simulink model "ChiefMaster_TTC580"  (R2022b)
settings: Solver=FixedStepAuto  StartTime=0.0  StopTime=10  FixedStep=0.01  RelTol=1e-3
values from neighbouring files (symbols this model uses):
  BattBox1_No = single(1)    [Parameters.m]
  BattBox2_No = single(2)    [Parameters.m]
  BattBox3_No = single(3)    [Parameters.m]
  CurrentLB = single(-3)    [Parameters.m]
  CurrentReductionConstant_Lvl0 = single(0.03)    [Parameters.m]
  CurrentReductionConstant_Lvl1 = single(0.05)    [Parameters.m]
  CurrentReductionConstant_Lvl2 = single(0.07)    [Parameters.m]
  CurrentReductionConstant_Lvl3 = single(0.1)    [Parameters.m]
  CurrentUB = single(3)    [Parameters.m]
  DCHV_Minus_In_Delay_ms = single(500)    [Parameters.m]
  FL_sHVC_CellBalanceVoltage_mV = single(3500)    [Parameters.m]
  FL_sInrushCurrent_dividebyzero = single(0.00001)    [Parameters.m]
  FL_u8HMI_BuzzerTimer = uint8(3)    [Parameters.m]
  IP_boActValue = true    [Parameters.m]
  IP_boDeactValue = false    [Parameters.m]
  IP_boInitValue = false    [Parameters.m]
  IP_s_LB = 18000    [Parameters.m]
  IP_s_UB = 22000    [Parameters.m]
  IP_sBatt1_ChargeCurrentMax_Factor = single(0.1)    [Parameters.m]
  IP_sBatt1_ChargeCurrentMax_LB = single(0)    [Parameters.m]
  IP_sBatt1_ChargeCurrentMax_Offset = single(0)    [Parameters.m]
  IP_sBatt1_ChargeCurrentMax_UB = single(6553.5)    [Parameters.m]
  IP_sBatt1_Current_Factor = single(0.1)    [Parameters.m]
  IP_sBatt1_Current_LB = single(-3276.8)    [Parameters.m]
  IP_sBatt1_Current_Offset = single(0)    [Parameters.m]
  IP_sBatt1_Current_UB = single(3276.8)    [Parameters.m]
  IP_sBatt1_DisChargeCurrentMax_Factor = single(0.1)    [Parameters.m]
  IP_sBatt1_DisChargeCurrentMax_LB = single(0)    [Parameters.m]
  IP_sBatt1_DisChargeCurrentMax_Offset = single(0)    [Parameters.m]
  IP_sBatt1_DisChargeCurrentMax_UB = single(6553.5)    [Parameters.m]
  IP_sBatt1_InsulationResistance_Factor = single(5)    [Parameters.m]
  IP_sBatt1_InsulationResistance_LB = single(0)    [Parameters.m]
  IP_sBatt1_InsulationResistance_Offset = single(0)    [Parameters.m]
  IP_sBatt1_InsulationResistance_UB = single(0)    [Parameters.m]
  IP_sBatt1_LiBa_IntResist_mOhm = single(25)    [Parameters.m]
  IP_sBatt1_SOC_Factor = single(1)    [Parameters.m]
  IP_sBatt1_SOC_LB = single(0)    [Parameters.m]
  IP_sBatt1_SOC_Offset = single(0)    [Parameters.m]
  IP_sBatt1_SOC_UB = single(100)    [Parameters.m]
  IP_sBatt1_SOH_Factor = single(1)    [Parameters.m]
  IP_sBatt1_SOH_LB = single(0)    [Parameters.m]
  IP_sBatt1_SOH_Offset = single(0)    [Parameters.m]
  IP_sBatt1_SOH_UB = single(100)    [Parameters.m]
  IP_sBatt1_Ubatt_Factor = single(0.1)    [Parameters.m]
  IP_sBatt1_Ubatt_LB = single(0)    [Parameters.m]
  IP_sBatt1_Ubatt_Offset = single(0)    [Parameters.m]
  IP_sBatt1_Ubatt_UB = single(6553.5)    [Parameters.m]
  IP_sBatt1_UserRi_Factor = single(1)    [Parameters.m]
  IP_sBatt1_UserRi_LB = single(0)    [Parameters.m]
  IP_sBatt1_UserRi_Offset = single(0)    [Parameters.m]
  IP_sBatt1_UserRi_UB = single(255)    [Parameters.m]
  IP_sBatt1_VoltageAtSensor_Factor = single(0.02)    [Parameters.m]
  IP_sBatt1_VoltageAtSensor_LB = single(0)    [Parameters.m]
  IP_sBatt1_VoltageAtSensor_Offset = single(0)    [Parameters.m]
  IP_sBatt1_VoltageAtSensor_UB = single(1310.7)    [Parameters.m]
  IP_sBatt2_LiBa_IntResist_mOhm = single(25)    [Parameters.m]
  IP_sBatt3_LiBa_IntResist_mOhm = single(25)    [Parameters.m]
  IP_sEM_LB = 2000    [Parameters.m]
  IP_sEM_UB = 8000    [Parameters.m]
  IP_sFB_LB = 5000    [Parameters.m]
  IP_sFB_UB = 10000    [Parameters.m]
  IP_sHVIL_LB = 12000    [Parameters.m]
  IP_sHVIL_UB = 15000    [Parameters.m]
  IP_sLoad_Voltage_Factor = single(1)    [Parameters.m]
  IP_sLoad_Voltage_LB = single(0)    [Parameters.m]
  IP_sLoad_Voltage_Offset = single(0)    [Parameters.m]
  IP_sLoad_Voltage_UB = single(65535)    [Parameters.m]
  IP_u8HVIL_Delay_ms = uint8(100)    [Parameters.m]
  IP_u8HW_IN_delay_ms = uint8(100)    [Parameters.m]
  IT_sInsulationSafeValue_kOhm = single(650)    [Parameters.m]
  IT_u8IMD_DelayTime_s = uint8(20)    [Parameters.m]
  MainHV_Minus_In_Delay = single(5)    [Parameters.m]
  MainHV_StatusDelay = single(5)    [Parameters.m]
  NotAvailable_uint16 = single(65535)    [Parameters.m]
  NotAvailable_uint8 = uint8(255)    [Parameters.m]
  OP_boHVIL_Supply = boolean(1)    [Parameters.m]
  SafeCurrentToCloseHV_A = single(5)    [Parameters.m]
  SafeVoltageToCloseHV_V = single(0.5)    [Parameters.m]
  UnexpectedBattChargingFcn_Available = boolean(1)    [Parameters.m]
  Voltage_NA_UB = uint16(65535)    [Parameters.m]
  VoltageSensorAvailableBB1 = boolean(0)    [Parameters.m]
  VoltageSensorAvailableBB2 = boolean(0)    [Parameters.m]
  VoltageSensorAvailableBB3 = boolean(0)    [Parameters.m]
libraries: simulink x184, Library_DataProcessing_v1_1 x167, Library_DataProcessing_v1 x142, libCM x28
(part 9 of 19)

== system ChiefMaster_TTC580/ChiefMaster/Output Processing/CM_OBD/CM_OP_Msg2 ==
  OT_Databus : Inport
  Bus Selector8 : BusSelector  OutputSignals=OT_KL15_Databus.OT_boKL15_BB1,OT_KL15_Databus.OT_boKL15_BB2,OT_KL15_Databus.OT_boKL15_BB3,OT_BDUControl_Databus.OT_boREQ_MainHV_ON_MINUS,OT_BDUControl_Databus.OT_boREQ_MainHV_ON_PLUS,OT_BDUControl_Databus.OT_boREQ_MainHV_ON_Precharge,OT_IMD_Databus.OT_boREQ_IMD_ON_BB1,OT_IMD_Databus.OT_boREQ_IMD_ON_BB2,OT_IMD_Databus.OT_boREQ_IMD_ON_BB3,OT_BatteryBox_HVControl_Databus.OT_boREQ_HV_ON_BB1,OT_BatteryBox_HVControl_Databus.OT_boREQ_HV_ON_BB2,OT_BatteryBox_HVControl_Databus.OT_boREQ_HV_ON_BB3,OT_BDUControl_Databus.OT_boREQ_DC_ON_MINUS,OT_BDUControl_Databus.OT_boREQ_DC_ON_Plus,OT_SystemStatus_Databus.OT_boSS_CabinAlarm,OT_SystemStatus_Databus.OT_boSS_EMSRET_POWER,OT_SystemStatus_Databus.OT_boSS_Resetbutton_LED
  Constant1 : Constant  Value=0  OutDataTypeStr=uint8
  Constant2 : Constant  Value=0  OutDataTypeStr=uint8
  Constant3 : Constant  Value=0  OutDataTypeStr=uint8
  Lib_MultiBit_Concat1 : Library_DataProcessing_v1/Lib_MultiBit_Concat  SystemSampleTime=-1  VariantActivationTime=update diagram  Latency=0  AutoFrameSizeCalculation=off
  Lib_MultiBit_Concat2 : Library_DataProcessing_v1/Lib_MultiBit_Concat  SystemSampleTime=-1  VariantActivationTime=update diagram  Latency=0  AutoFrameSizeCalculation=off
  Lib_MultiBit_Concat7 : Library_DataProcessing_v1/Lib_MultiBit_Concat  SystemSampleTime=-1  VariantActivationTime=update diagram  Latency=0  AutoFrameSizeCalculation=off
  Mux : Mux  Inputs=8
  OP_ChiefMaster_OP_Msg2 : Outport
  wires:
  OT_Databus/1 -> Bus Selector8/1
  Lib_MultiBit_Concat7/1 -> Mux/1
  Bus Selector8/1 -> Lib_MultiBit_Concat7/1  "<OT_boKL15_BB1>"
  Bus Selector8/2 -> Lib_MultiBit_Concat7/2  "<OT_boKL15_BB2>"
  Bus Selector8/3 -> Lib_MultiBit_Concat7/3  "<OT_boKL15_BB3>"
  Bus Selector8/4 -> Lib_MultiBit_Concat7/4  "<OT_boREQ_MainHV_ON_MINUS>"
  Bus Selector8/5 -> Lib_MultiBit_Concat7/5  "<OT_boREQ_MainHV_ON_PLUS>"
  Bus Selector8/6 -> Lib_MultiBit_Concat7/6  "<OT_boREQ_MainHV_ON_Precharge>"
  Constant2/1 -> Mux/7, Mux/6, Mux/4, Mux/5, Mux/8
  Mux/1 -> OP_ChiefMaster_OP_Msg2/1
  Bus Selector8/7 -> Lib_MultiBit_Concat7/7  "<OT_boREQ_IMD_ON_BB1>"
  Bus Selector8/8 -> Lib_MultiBit_Concat7/8  "<OT_boREQ_IMD_ON_BB2>"
  Bus Selector8/9 -> Lib_MultiBit_Concat1/1  "<OT_boREQ_IMD_ON_BB3>"
  Bus Selector8/10 -> Lib_MultiBit_Concat1/2  "<OT_boREQ_HV_ON_BB1>"
  Bus Selector8/11 -> Lib_MultiBit_Concat1/3  "<OT_boREQ_HV_ON_BB2>"
  Bus Selector8/12 -> Lib_MultiBit_Concat1/4  "<OT_boREQ_HV_ON_BB3>"
  Lib_MultiBit_Concat1/1 -> Mux/2
  Bus Selector8/13 -> Lib_MultiBit_Concat1/5  "<OT_boREQ_DC_ON_MINUS>"
  Bus Selector8/14 -> Lib_MultiBit_Concat1/6  "<OT_boREQ_DC_ON_Plus>"
  Bus Selector8/15 -> Lib_MultiBit_Concat2/1  "<OT_boSS_CabinAlarm>"
  Bus Selector8/16 -> Lib_MultiBit_Concat2/2  "<OT_boSS_EMSRET_POWER>"
  Bus Selector8/17 -> Lib_MultiBit_Concat2/3  "<OT_boSS_Resetbutton_LED>"
  Constant1/1 -> Lib_MultiBit_Concat1/7, Lib_MultiBit_Concat1/8
  Constant3/1 -> Lib_MultiBit_Concat2/8, Lib_MultiBit_Concat2/6, Lib_MultiBit_Concat2/4, Lib_MultiBit_Concat2/5, Lib_MultiBit_Concat2/7
  Lib_MultiBit_Concat2/1 -> Mux/3

== system ChiefMaster_TTC580/ChiefMaster/Output Processing/CM_OBD/CM_SystemStatus1_Msg3 ==
  OT_Databus : Inport
  Bus Selector3 : BusSelector  OutputSignals=OT_boCM_Sleep,OT_SystemStatus_Databus.OT_boSS_HVIL_NOK,OT_SystemStatus_Databus.OT_u8SS_ChiefMaster_State,OT_SystemStatus_Databus.OT_u8SS_System_ErrorCode,OT_SystemStatus_Databus.OT_u8SS_System_SD_ErrorCode,OT_SystemStatus_Databus.OT_u8SS_SystemSOC,OT_IMD_Databus.OT_u8_IMD_State_BB1,OT_IMD_Databus.OT_u8_IMD_State_BB2,OT_IMD_Databus.OT_u8_IMD_State_BB3
  Bus Selector5 : BusSelector  OutputSignals=OT_SystemStatus_Databus.OT_boSS_Batt_Warning,OT_SystemStatus_Databus.OT_boSS_Batt_Error,OT_SystemStatus_Databus.OT_boSS_Batt_SDError,OT_SystemStatus_Databus.OT_boSS_System_Error,OT_SystemStatus_Databus.OT_boSS_System_SD,OT_SystemStatus_Databus.OT_boSS_System_ESD,OT_SystemStatus_Databus.OT_boSS_BDU_Reset,FL_Databus.FL_KL15_Databus.FL_boKL15_Disable,FL_Databus.FL_KL15_Databus.FL_boKL15_Reset,FL_Databus.IT_Databus.IT_BatterySignal_Databus.IT_boBMS_HV_ON_BB,FL_Databus.IT_Databus.IT_BatterySignal_Databus.IT_u8BMS_No_of_Battery_Usable,OT_SystemStatus_Databus.OT_u8SS_NumberOfConnectedBatt,OT_SystemStatus_Databus.OT_u8SS_EmergencyStopState
  Constant1 : Constant  Value=0  OutDataTypeStr=uint8
  Constant4 : Constant  Value=0  OutDataTypeStr=uint8
  Extract Bits1 : simulink/Logic and Bit Operations/Extract Bits  bitsToExtract=Range of bits  numBits=8  bitIdxRange=[0 1]  outScalingMode=Treat bit field as an integer
  Extract Bits2 : simulink/Logic and Bit Operations/Extract Bits  bitsToExtract=Range of bits  numBits=8  bitIdxRange=[0 1]  outScalingMode=Treat bit field as an integer
  Extract Bits3 : simulink/Logic and Bit Operations/Extract Bits  bitsToExtract=Range of bits  numBits=8  bitIdxRange=[0 1]  outScalingMode=Treat bit field as an integer
  Extract Bits4 : simulink/Logic and Bit Operations/Extract Bits  bitsToExtract=Range of bits  numBits=8  bitIdxRange=[0 2]  outScalingMode=Treat bit field as an integer
  Extract Bits5 : simulink/Logic and Bit Operations/Extract Bits  bitsToExtract=Range of bits  numBits=8  bitIdxRange=[0 2]  outScalingMode=Treat bit field as an integer
  Extract Bits6 : simulink/Logic and Bit Operations/Extract Bits  bitsToExtract=Range of bits  numBits=8  bitIdxRange=[0 2]  outScalingMode=Treat bit field as an integer
  Lib_MultiBit_Concat{1..4} (4 alike) : Library_DataProcessing_v1/Lib_MultiBit_Concat  SystemSampleTime=-1  VariantActivationTime=update diagram  Latency=0  AutoFrameSizeCalculation=off
  Mux : Mux  Inputs=8
  Subsystem : Subsystem
  OP_ChiefMaster_SS_Msg3 : Outport
  wires:
  Mux/1 -> OP_ChiefMaster_SS_Msg3/1
  Bus Selector5/1 -> Lib_MultiBit_Concat1/1  "<OT_boSS_Batt_Warning>"
  Bus Selector5/2 -> Lib_MultiBit_Concat1/2  "<OT_boSS_Batt_Error>"
  Bus Selector5/3 -> Lib_MultiBit_Concat1/3  "<OT_boSS_Batt_SDError>"
  Bus Selector5/4 -> Lib_MultiBit_Concat1/4  "<OT_boSS_System_Error>"
  Bus Selector5/5 -> Lib_MultiBit_Concat1/5  "<OT_boSS_System_SD>"
  Bus Selector5/6 -> Lib_MultiBit_Concat1/6  "<OT_boSS_System_ESD>"
  Bus Selector5/7 -> Lib_MultiBit_Concat1/7  "<OT_boSS_BDU_Reset>"
  Bus Selector5/12 -> Extract Bits3/1  "<OT_u8SS_NumberOfConnectedBatt>"
  Bus Selector5/13 -> Extract Bits2/1  "<OT_u8SS_EmergencyStopState>"
  Constant4/1 -> Lib_MultiBit_Concat2/6, Lib_MultiBit_Concat2/4, Lib_MultiBit_Concat2/8, Lib_MultiBit_Concat3/4, Lib_MultiBit_Concat3/5, Lib_MultiBit_Concat3/7, Lib_MultiBit_Concat3/8
  Bus Selector5/8 -> Lib_MultiBit_Concat1/8  "<FL_boKL15_Disable>"
  Bus Selector5/9 -> Lib_MultiBit_Concat2/1  "<FL_boKL15_Reset>"
  Lib_MultiBit_Concat1/1 -> Mux/1
  Lib_MultiBit_Concat2/1 -> Mux/2
  Bus Selector5/10 -> Lib_MultiBit_Concat2/2  "<IT_boBMS_HV_ON_BB>"
  Bus Selector5/11 -> Extract Bits1/1  "<IT_u8BMS_No_of_Battery_Usable>"
  Extract Bits1/1 -> Lib_MultiBit_Concat2/3
  Extract Bits3/1 -> Lib_MultiBit_Concat2/5
  Extract Bits2/1 -> Lib_MultiBit_Concat2/7
  Lib_MultiBit_Concat4/1 -> Mux/8
  Bus Selector3/1 -> Lib_MultiBit_Concat3/1  "<OT_boCM_Sleep>"
  Bus Selector3/3 -> Mux/4  "<OT_u8SS_ChiefMaster_State>"
  Lib_MultiBit_Concat3/1 -> Mux/3
  Bus Selector3/4 -> Mux/5  "<OT_u8SS_System_ErrorCode>"
  Bus Selector3/5 -> Mux/6  "<OT_u8SS_System_SD_ErrorCode>"
  Bus Selector3/6 -> Mux/7  "<OT_u8SS_SystemSOC>"
  Bus Selector3/2 -> Lib_MultiBit_Concat3/2  "<OT_boSS_HVIL_NOK>"
  OT_Databus/1 -> Bus Selector5/1, Subsystem/1(IP_DataBus), Bus Selector3/1
  Subsystem/1(FL_boHVC_AllCellBalanced) -> Lib_MultiBit_Concat3/3
  Bus Selector3/7 -> Extract Bits4/1  "<OT_u8_IMD_State_BB1>"
  Bus Selector3/8 -> Extract Bits5/1  "<OT_u8_IMD_State_BB2>"
  Bus Selector3/9 -> Extract Bits6/1  "<OT_u8_IMD_State_BB3>"
  Extract Bits4/1 -> Lib_MultiBit_Concat3/6
  Extract Bits5/1 -> Lib_MultiBit_Concat4/1
  Extract Bits6/1 -> Lib_MultiBit_Concat4/4
  Constant1/1 -> Lib_MultiBit_Concat4/8, Lib_MultiBit_Concat4/7, Lib_MultiBit_Concat4/2, Lib_MultiBit_Concat4/3, Lib_MultiBit_Concat4/5, Lib_MultiBit_Concat4/6

== system ChiefMaster_TTC580/ChiefMaster/Output Processing/CM_OBD/CM_SystemStatus2_Msg4 ==
  OT_Databus : Inport
  Bus Selector3 : BusSelector  OutputSignals=OT_SystemStatus_Databus.OT_sSS_System_Current,OT_SystemStatus_Databus.OT_sSS_SystemVoltage,OT_SystemStatus_Databus.OT_sSS_MaxChargeCurrent,OT_SystemStatus_Databus.OT_sSS_MaxDisChargeCurrent
  Mux1 : Mux  Inputs=8
  Subsystem : Subsystem
  Subsystem1 : Subsystem
  Subsystem2 : Subsystem
  Subsystem3 : Subsystem
  OP_ChiefMaster_SS2_Msg4 : Outport
  wires:
  Subsystem1/1(u8byte_LSB) -> Mux1/3
  Subsystem2/1(u8byte_LSB) -> Mux1/5
  Bus Selector3/4 -> Subsystem3/1(MaxDisChargeCurrent)  "<OT_sSS_MaxDisChargeCurrent>"
  Bus Selector3/1 -> Subsystem/1(System_Current)  "<OT_sSS_System_Current>"
  Subsystem/2(u8byte_MSB) -> Mux1/2
  Subsystem2/2(u8byte_MSB) -> Mux1/6
  Bus Selector3/2 -> Subsystem1/1(System_Voltage)  "<OT_sSS_SystemVoltage>"
  Mux1/1 -> OP_ChiefMaster_SS2_Msg4/1
  Subsystem1/2(u8byte_MSB) -> Mux1/4
  Subsystem3/1(u8byte_LSB) -> Mux1/7
  Bus Selector3/3 -> Subsystem2/1(MaxChargeCurrent)  "<OT_sSS_MaxChargeCurrent>"
  Subsystem3/2(u8byte_MSB) -> Mux1/8
  Subsystem/1(u8byte_LSB) -> Mux1/1
  OT_Databus/1 -> Bus Selector3/1

== system ChiefMaster_TTC580/ChiefMaster/Output Processing/OP_Actia/Subsystem2 ==
  <FL_boREQ_HV_ON_BB1> : Inport
  <FL_boREQ_IMD_ON_BB1> : Inport  Port=2
  Constant15 : Constant  Priority=2915  Value=0
  Constant3 : Constant  Priority=2915  Value=0  OutDataTypeStr=uint8
  Lib_MultiBit_Concat1 : Library_DataProcessing_v1/Lib_MultiBit_Concat  SystemSampleTime=-1  VariantActivationTime=update diagram  Latency=0  AutoFrameSizeCalculation=off
  Mux : Mux  Inputs=8
  OP_Actia_Control_Batt1 : Outport
  wires:
  Constant3/1 -> Mux/7, Mux/6, Mux/5, Mux/4, Mux/3, Mux/2, Mux/8
  Constant15/1 -> Lib_MultiBit_Concat1/7, Lib_MultiBit_Concat1/5, Lib_MultiBit_Concat1/3, Lib_MultiBit_Concat1/4, Lib_MultiBit_Concat1/6, Lib_MultiBit_Concat1/8
  <FL_boREQ_HV_ON_BB1>/1 -> Lib_MultiBit_Concat1/1
  Lib_MultiBit_Concat1/1 -> Mux/1
  Mux/1 -> OP_Actia_Control_Batt1/1
  <FL_boREQ_IMD_ON_BB1>/1 -> Lib_MultiBit_Concat1/2

== system ChiefMaster_TTC580/ChiefMaster/Output Processing/OP_Actia/Subsystem3 ==
  <FL_boREQ_HV_ON_BB2> : Inport
  <FL_boREQ_IMD_ON_BB2> : Inport  Port=2
  Constant1 : Constant  Priority=2915  Value=0
  Constant4 : Constant  Priority=2915  Value=0  OutDataTypeStr=uint8
  Lib_MultiBit_Concat2 : Library_DataProcessing_v1/Lib_MultiBit_Concat  SystemSampleTime=-1  VariantActivationTime=update diagram  Latency=0  AutoFrameSizeCalculation=off
  Mux1 : Mux  Inputs=8
  OP_Actia_Control_Batt2 : Outport
  wires:
  Constant4/1 -> Mux1/8, Mux1/2, Mux1/3, Mux1/4, Mux1/5, Mux1/6, Mux1/7
  Constant1/1 -> Lib_MultiBit_Concat2/8, Lib_MultiBit_Concat2/6, Lib_MultiBit_Concat2/4, Lib_MultiBit_Concat2/3, Lib_MultiBit_Concat2/5, Lib_MultiBit_Concat2/7
  <FL_boREQ_IMD_ON_BB2>/1 -> Lib_MultiBit_Concat2/2
  Lib_MultiBit_Concat2/1 -> Mux1/1
  Mux1/1 -> OP_Actia_Control_Batt2/1
  <FL_boREQ_HV_ON_BB2>/1 -> Lib_MultiBit_Concat2/1

== system ChiefMaster_TTC580/ChiefMaster/Output Processing/OP_Actia/Subsystem4 ==
  <FL_boREQ_HV_ON_BB3> : Inport
  <FL_boREQ_IMD_ON_BB3> : Inport  Port=2
  Constant2 : Constant  Priority=2915  Value=0
  Constant5 : Constant  Priority=2915  Value=0  OutDataTypeStr=uint8
  Lib_MultiBit_Concat3 : Library_DataProcessing_v1/Lib_MultiBit_Concat  SystemSampleTime=-1  VariantActivationTime=update diagram  Latency=0  AutoFrameSizeCalculation=off
  Mux2 : Mux  Inputs=8
  OP_Actia_Control_Batt3 : Outport
  wires:
  <FL_boREQ_IMD_ON_BB3>/1 -> Lib_MultiBit_Concat3/2
  Constant2/1 -> Lib_MultiBit_Concat3/7, Lib_MultiBit_Concat3/5, Lib_MultiBit_Concat3/3, Lib_MultiBit_Concat3/4, Lib_MultiBit_Concat3/6, Lib_MultiBit_Concat3/8
  Constant5/1 -> Mux2/7, Mux2/6, Mux2/5, Mux2/4, Mux2/3, Mux2/2, Mux2/8
  <FL_boREQ_HV_ON_BB3>/1 -> Lib_MultiBit_Concat3/1
  Mux2/1 -> OP_Actia_Control_Batt3/1
  Lib_MultiBit_Concat3/1 -> Mux2/1

== system ChiefMaster_TTC580/ChiefMaster/Output Processing/OP_LiBa/UDC_BMS_OperationRequest1 ==
  OT_Databus : Inport
  Bus Selector1 : BusSelector  OutputSignals=OT_BatteryBox_HVControl_Databus.OT_boREQ_HV_ON_BB1,OT_IMD_Databus.OT_boREQ_IMD_ON_BB1
  Constant{,1..4} (5 alike) : Constant  Value=0  OutDataTypeStr=uint8
  Constant5 : Constant  OutDataTypeStr=uint8
  Data Type Conversion : DataTypeConversion  OutDataTypeStr=uint8  RndMeth=Nearest  SaturateOnIntegerOverflow=off
  Data Type Conversion1 : DataTypeConversion  OutDataTypeStr=uint8  RndMeth=Nearest  SaturateOnIntegerOverflow=off
  Data Type Conversion2 : DataTypeConversion  OutDataTypeStr=uint16  RndMeth=Nearest  SaturateOnIntegerOverflow=off
  Extract Bits : simulink/Logic and Bit Operations/Extract Bits  bitsToExtract=Range of bits  numBits=8  bitIdxRange=[0 1]  outScalingMode=Preserve fixed-point scaling
  Extract Bits1 : simulink/Logic and Bit Operations/Extract Bits  bitsToExtract=Range of bits  numBits=8  bitIdxRange=[0 1]  outScalingMode=Preserve fixed-point scaling
  Extract Bits2 : simulink/Logic and Bit Operations/Extract Bits  bitsToExtract=Range of bits  numBits=8  bitIdxRange=[0 1]  outScalingMode=Preserve fixed-point scaling
  Extract Bits3 : simulink/Logic and Bit Operations/Extract Bits  bitsToExtract=Range of bits  numBits=8  bitIdxRange=[0 7]  outScalingMode=Treat bit field as an integer
  Extract Bits4 : simulink/Logic and Bit Operations/Extract Bits  bitsToExtract=Range of bits  numBits=8  bitIdxRange=[8 15]  outScalingMode=Treat bit field as an integer
  Lib_MultiBit_Concat : Library_DataProcessing_v1_1/Lib_MultiBit_Concat  SystemSampleTime=-1  VariantActivationTime=update diagram  Latency=0  AutoFrameSizeCalculation=off
  Mux : Mux  Inputs=8
  OP_UDC_BMS_OperationRequest : Outport
  wires:
  Mux/1 -> OP_UDC_BMS_OperationRequest/1
  Lib_MultiBit_Concat/1 -> Mux/1
  Constant/1 -> Mux/8, Mux/7, Mux/6, Mux/5, Mux/4
  OT_Databus/1 -> Bus Selector1/1
  Extract Bits/1 -> Lib_MultiBit_Concat/1
  Extract Bits1/1 -> Lib_MultiBit_Concat/3
  Extract Bits2/1 -> Lib_MultiBit_Concat/7
  Constant1/1 -> Lib_MultiBit_Concat/2
  Constant2/1 -> Lib_MultiBit_Concat/6, Lib_MultiBit_Concat/5, Lib_MultiBit_Concat/4
  Constant3/1 -> Lib_MultiBit_Concat/8
  Constant4/1 -> Extract Bits/1
  Constant5/1 -> Extract Bits2/1
  Data Type Conversion/1 -> Mux/2
  Data Type Conversion1/1 -> Mux/3
  Extract Bits4/1 -> Data Type Conversion1/1
  Extract Bits3/1 -> Data Type Conversion/1
  Data Type Conversion2/1 -> Extract Bits4/1, Extract Bits3/1
  Bus Selector1/1 -> Extract Bits1/1  "<OT_boREQ_HV_ON_BB1>"
  Bus Selector1/2 -> Data Type Conversion2/1  "<OT_boREQ_IMD_ON_BB1>"

== system ChiefMaster_TTC580/ChiefMaster/Output Processing/OP_LiBa/UDC_BMS_OperationRequest2 ==
  OT_Databus : Inport
  Bus Selector1 : BusSelector  OutputSignals=OT_BatteryBox_HVControl_Databus.OT_boREQ_HV_ON_BB2,OT_IMD_Databus.OT_boREQ_IMD_ON_BB2
  Constant{,1..4} (5 alike) : Constant  Value=0  OutDataTypeStr=uint8
  Constant5 : Constant  OutDataTypeStr=uint8
  Data Type Conversion : DataTypeConversion  OutDataTypeStr=uint8  RndMeth=Nearest  SaturateOnIntegerOverflow=off
  Data Type Conversion1 : DataTypeConversion  OutDataTypeStr=uint8  RndMeth=Nearest  SaturateOnIntegerOverflow=off
  Data Type Conversion2 : DataTypeConversion  OutDataTypeStr=uint16  RndMeth=Nearest  SaturateOnIntegerOverflow=off
  Extract Bits : simulink/Logic and Bit Operations/Extract Bits  bitsToExtract=Range of bits  numBits=8  bitIdxRange=[0 1]  outScalingMode=Preserve fixed-point scaling
  Extract Bits1 : simulink/Logic and Bit Operations/Extract Bits  bitsToExtract=Range of bits  numBits=8  bitIdxRange=[0 1]  outScalingMode=Preserve fixed-point scaling
  Extract Bits2 : simulink/Logic and Bit Operations/Extract Bits  bitsToExtract=Range of bits  numBits=8  bitIdxRange=[0 1]  outScalingMode=Preserve fixed-point scaling
  Extract Bits3 : simulink/Logic and Bit Operations/Extract Bits  bitsToExtract=Range of bits  numBits=8  bitIdxRange=[0 7]  outScalingMode=Treat bit field as an integer
  Extract Bits4 : simulink/Logic and Bit Operations/Extract Bits  bitsToExtract=Range of bits  numBits=8  bitIdxRange=[8 15]  outScalingMode=Treat bit field as an integer
  Lib_MultiBit_Concat : Library_DataProcessing_v1_1/Lib_MultiBit_Concat  SystemSampleTime=-1  VariantActivationTime=update diagram  Latency=0  AutoFrameSizeCalculation=off
  Mux : Mux  Inputs=8
  OP_UDC_BMS_OperationRequest : Outport
  wires:
  Bus Selector1/2 -> Data Type Conversion2/1  "<OT_boREQ_IMD_ON_BB2>"
  Bus Selector1/1 -> Extract Bits1/1  "<OT_boREQ_HV_ON_BB2>"
  Data Type Conversion2/1 -> Extract Bits3/1, Extract Bits4/1
  Extract Bits3/1 -> Data Type Conversion/1
  Extract Bits4/1 -> Data Type Conversion1/1
  Data Type Conversion1/1 -> Mux/3
  Data Type Conversion/1 -> Mux/2
  Constant5/1 -> Extract Bits2/1
  Constant4/1 -> Extract Bits/1
  Constant3/1 -> Lib_MultiBit_Concat/8
  Constant2/1 -> Lib_MultiBit_Concat/4, Lib_MultiBit_Concat/5, Lib_MultiBit_Concat/6
  Constant1/1 -> Lib_MultiBit_Concat/2
  Extract Bits2/1 -> Lib_MultiBit_Concat/7
  Extract Bits1/1 -> Lib_MultiBit_Concat/3
  Extract Bits/1 -> Lib_MultiBit_Concat/1
  OT_Databus/1 -> Bus Selector1/1
  Constant/1 -> Mux/4, Mux/5, Mux/6, Mux/7, Mux/8
  Lib_MultiBit_Concat/1 -> Mux/1
  Mux/1 -> OP_UDC_BMS_OperationRequest/1

== system ChiefMaster_TTC580/ChiefMaster/Output Processing/OP_LiBa/UDC_BMS_OperationRequest3 ==
  OT_Databus : Inport
  Bus Selector1 : BusSelector  OutputSignals=OT_BatteryBox_HVControl_Databus.OT_boREQ_HV_ON_BB3,OT_IMD_Databus.OT_boREQ_IMD_ON_BB3
  Constant{,1..4} (5 alike) : Constant  Value=0  OutDataTypeStr=uint8
  Constant5 : Constant  OutDataTypeStr=uint8
  Data Type Conversion : DataTypeConversion  OutDataTypeStr=uint8  RndMeth=Nearest  SaturateOnIntegerOverflow=off
  Data Type Conversion1 : DataTypeConversion  OutDataTypeStr=uint8  RndMeth=Nearest  SaturateOnIntegerOverflow=off
  Data Type Conversion2 : DataTypeConversion  OutDataTypeStr=uint16  RndMeth=Nearest  SaturateOnIntegerOverflow=off
  Extract Bits : simulink/Logic and Bit Operations/Extract Bits  bitsToExtract=Range of bits  numBits=8  bitIdxRange=[0 1]  outScalingMode=Preserve fixed-point scaling
  Extract Bits1 : simulink/Logic and Bit Operations/Extract Bits  bitsToExtract=Range of bits  numBits=8  bitIdxRange=[0 1]  outScalingMode=Preserve fixed-point scaling
  Extract Bits2 : simulink/Logic and Bit Operations/Extract Bits  bitsToExtract=Range of bits  numBits=8  bitIdxRange=[0 1]  outScalingMode=Preserve fixed-point scaling
  Extract Bits3 : simulink/Logic and Bit Operations/Extract Bits  bitsToExtract=Range of bits  numBits=8  bitIdxRange=[0 7]  outScalingMode=Treat bit field as an integer
  Extract Bits4 : simulink/Logic and Bit Operations/Extract Bits  bitsToExtract=Range of bits  numBits=8  bitIdxRange=[8 15]  outScalingMode=Treat bit field as an integer
  Lib_MultiBit_Concat : Library_DataProcessing_v1_1/Lib_MultiBit_Concat  SystemSampleTime=-1  VariantActivationTime=update diagram  Latency=0  AutoFrameSizeCalculation=off
  Mux : Mux  Inputs=8
  OP_UDC_BMS_OperationRequest : Outport
  wires:
  Mux/1 -> OP_UDC_BMS_OperationRequest/1
  Lib_MultiBit_Concat/1 -> Mux/1
  Constant/1 -> Mux/8, Mux/7, Mux/6, Mux/5, Mux/4
  OT_Databus/1 -> Bus Selector1/1
  Extract Bits/1 -> Lib_MultiBit_Concat/1
  Extract Bits1/1 -> Lib_MultiBit_Concat/3
  Extract Bits2/1 -> Lib_MultiBit_Concat/7
  Constant1/1 -> Lib_MultiBit_Concat/2
  Constant2/1 -> Lib_MultiBit_Concat/6, Lib_MultiBit_Concat/5, Lib_MultiBit_Concat/4
  Constant3/1 -> Lib_MultiBit_Concat/8
  Constant4/1 -> Extract Bits/1
  Constant5/1 -> Extract Bits2/1
  Data Type Conversion/1 -> Mux/2
  Data Type Conversion1/1 -> Mux/3
  Extract Bits4/1 -> Data Type Conversion1/1
  Extract Bits3/1 -> Data Type Conversion/1
  Data Type Conversion2/1 -> Extract Bits4/1, Extract Bits3/1
  Bus Selector1/1 -> Extract Bits1/1  "<OT_boREQ_HV_ON_BB3>"
  Bus Selector1/2 -> Data Type Conversion2/1  "<OT_boREQ_IMD_ON_BB3>"

== system ChiefMaster_TTC580/ChiefMaster/Output Translation/IMD/Subsystem ==
  <FL_boREQ_IMD_ON_BB1> : Inport
  Constant : Constant  Value=0  OutDataTypeStr=boolean
  Multiport Switch : MultiPortSwitch  DataPortForDefault=Additional data port  DiagnosticForDefault=Warning  SaturateOnIntegerOverflow=off  InputSameDT=off
  OT_boREQ_IMD_ON_BB1 : Outport
  wires:
  Multiport Switch/1 -> OT_boREQ_IMD_ON_BB1/1  "OT_boREQ_IMD_ON_BB1"
  [Select_Battery1] -> Multiport Switch/1
  Constant/1 -> Multiport Switch/4, Multiport Switch/5
  <FL_boREQ_IMD_ON_BB1>/1 -> Multiport Switch/3, Multiport Switch/2

== system ChiefMaster_TTC580/ChiefMaster/Output Translation/IMD/Subsystem1 ==
  <FL_boREQ_IMD_ON_BB2> : Inport
  Constant : Constant  Value=0  OutDataTypeStr=boolean
  Multiport Switch : MultiPortSwitch  DataPortForDefault=Additional data port  DiagnosticForDefault=Warning  SaturateOnIntegerOverflow=off  InputSameDT=off
  OT_boREQ_IMD_ON_BB2 : Outport
  wires:
  <FL_boREQ_IMD_ON_BB2>/1 -> Multiport Switch/3, Multiport Switch/2
  Constant/1 -> Multiport Switch/5, Multiport Switch/4
  [Select_Battery2] -> Multiport Switch/1
  Multiport Switch/1 -> OT_boREQ_IMD_ON_BB2/1  "OT_boREQ_IMD_ON_BB2"

== system ChiefMaster_TTC580/ChiefMaster/Output Translation/IMD/Subsystem2 ==
  <FL_boREQ_IMD_ON_BB3> : Inport
  Constant : Constant  Value=0  OutDataTypeStr=boolean
  Multiport Switch : MultiPortSwitch  DataPortForDefault=Additional data port  DiagnosticForDefault=Warning  SaturateOnIntegerOverflow=off  InputSameDT=off
  OT_boREQ_IMD_ON_BB3 : Outport
  wires:
  Multiport Switch/1 -> OT_boREQ_IMD_ON_BB3/1  "OT_boREQ_IMD_ON_BB3"
  [Select_Battery3] -> Multiport Switch/1
  Constant/1 -> Multiport Switch/4, Multiport Switch/5
  <FL_boREQ_IMD_ON_BB3>/1 -> Multiport Switch/3, Multiport Switch/2

== system ChiefMaster_TTC580/ChiefMaster/Flow Logic/BDU Control/BDUSystem/Subsystem ==
  MainHV_ON_Plus_FB : Inport
  MainHV_ON_Minus_FB : Inport  Port=2
  FL_boCMSleep : Inport  Port=3
  FL_boREQ_MainHV_ON_MINUS : Inport  Port=4
  FL_boREQ_MainHV_ON_PLUS : Inport  Port=5
  Chart_Main_MinMAx_Status : libCM/Chart_Main_MinMAx_Status  SystemSampleTime=-1  VariantActivationTime=update diagram  Latency=0  AutoFrameSizeCalculation=off
      settings: PortSchema="{\"entries\":[{\"content\":{\"sides\":[{\"content\":{\"connectorIds\":[\"In1\",\"In2\",\"In4\",\"In3\"]},\"type\":\"ConnectorPlacement.EquallySpacedRectSide\",\"uuid\":\"af513ad7-882d-44ca-bd16-f13375ad0cc7\"},{\"content\":{\"connectorIds\":[\"Out1\"],\"side\":\"RIGHT\"},\"type\":\"ConnectorPlacement.EquallySpacedRectSide\",\"uuid\":\"1e07241b-ff1c-4b1c-99ea-8f556d1f4bde\"},{\"content\":{\"connectorIds\":[],\"side\":\"TOP\"},\"type\":\"ConnectorPlacement.EquallySpacedRectSide\",\"uuid\":\"c2fbf455-7245-4f9b-917b-4eed34a267cf\"}]},\"type\":\"ConnectorPlacement.EquallySpacedConnector\",\"uuid\":\"56193be1-d801-449e-8417-1819ff958dca\"}],\"packageUris\":[\"http://schema.mathworks.com/mf0/Connector/R2020b\"],\"version\":\"1.0\"}"
  Chart_Main_MinMAx_Status1 : libCM/Chart_Main_MinMAx_Status  SystemSampleTime=-1  VariantActivationTime=update diagram  Latency=0  AutoFrameSizeCalculation=off
      settings: PortSchema="{\"entries\":[{\"content\":{\"sides\":[{\"content\":{\"connectorIds\":[\"In1\",\"In2\",\"In4\",\"In3\"]},\"type\":\"ConnectorPlacement.EquallySpacedRectSide\",\"uuid\":\"af513ad7-882d-44ca-bd16-f13375ad0cc7\"},{\"content\":{\"connectorIds\":[\"Out1\"],\"side\":\"RIGHT\"},\"type\":\"ConnectorPlacement.EquallySpacedRectSide\",\"uuid\":\"1e07241b-ff1c-4b1c-99ea-8f556d1f4bde\"},{\"content\":{\"connectorIds\":[],\"side\":\"TOP\"},\"type\":\"ConnectorPlacement.EquallySpacedRectSide\",\"uuid\":\"c2fbf455-7245-4f9b-917b-4eed34a267cf\"}]},\"type\":\"ConnectorPlacement.EquallySpacedConnector\",\"uuid\":\"56193be1-d801-449e-8417-1819ff958dca\"}],\"packageUris\":[\"http://schema.mathworks.com/mf0/Connector/R2020b\"],\"version\":\"1.0\"}"
  Constant2 : Constant  Value=MainHV_StatusDelay
  FL_u8MainHV_Minus_Status : Outport
  FL_u8MainHV_Plus_Status : Outport  Port=2
  wires:
  FL_boREQ_MainHV_ON_MINUS/1 -> Chart_Main_MinMAx_Status1/1  "REQ_MainHV_ON_MINUS"
  Chart_Main_MinMAx_Status1/1 -> FL_u8MainHV_Minus_Status/1  "FL_u8MainHV_Minus_Status"
  MainHV_ON_Minus_FB/1 -> Chart_Main_MinMAx_Status1/2  "MainHV_ON_Minus_FB"
  MainHV_ON_Plus_FB/1 -> Chart_Main_MinMAx_Status/2  "MainHV_ON_Plus_FB"
  Chart_Main_MinMAx_Status/1 -> FL_u8MainHV_Plus_Status/1  "FL_u8MainHV_Plus_Status"
  FL_boREQ_MainHV_ON_PLUS/1 -> Chart_Main_MinMAx_Status/1  "REQ_MainHV_ON_PLUS"
  Constant2/1 -> Chart_Main_MinMAx_Status1/3, Chart_Main_MinMAx_Status/3
  FL_boCMSleep/1 -> Chart_Main_MinMAx_Status1/4, Chart_Main_MinMAx_Status/4

== system ChiefMaster_TTC580/ChiefMaster/Flow Logic/BDU Control/BDUSystem/Subsystem1 ==
  REQ_MainHV_ON_MINUS : Inport
  KL15_CM_Disable : Inport  Port=2
  WeldingDetection_Status : Inport  Port=3
  AND3 : Logic  AllPortsSameDT=off  OutDataTypeStr=boolean
  Chart4 : Stateflow chart
  Detect Decrease : simulink/Logic and Bit Operations/Detect Decrease  vinit=0.0  OutDataTypeStr=boolean
  Unit Delay : UnitDelay  SampleTime=-1  HasFrameUpgradeWarning=on
  FL_boMainHV_WeldingCheckEnable : Outport
  FL_boMainHV_WeldingCheckActive : Outport  Port=2
  wires:
  KL15_CM_Disable/1 -> AND3/2
  Chart4/1(Out) -> FL_boMainHV_WeldingCheckActive/1
  AND3/1 -> FL_boMainHV_WeldingCheckEnable/1, Chart4/1(In)
  REQ_MainHV_ON_MINUS/1 -> Detect Decrease/1
  Detect Decrease/1 -> AND3/1
  WeldingDetection_Status/1 -> Unit Delay/1
  Unit Delay/1 -> Chart4/2(WeldingDetection_Status)

== system ChiefMaster_TTC580/ChiefMaster/Flow Logic/BDU Control/BDUSystem/Subsystem2 ==
  SystemVtg : Inport
  LoadVtg : Inport  Port=2
  FL_boMainHV_WeldingCheckEnable : Inport  Port=3
  Chart_WeldingDetection : Stateflow chart  TreatAsAtomicUnit=on
      settings: RTWSystemCode=Reusable function  RTWFcnNameOpts=Use subsystem name  RTWFileNameOpts=Use subsystem name  PortSchema="{\"entries\":[{\"content\":{\"sides\":[{\"content\":{\"connectorIds\":[\"In2\",\"In1\",\"In3\"]},\"type\":\"ConnectorPlacement.EquallySpacedRectSide\",\"uuid\":\"8b7305c9-c54a-4462-8eb5-bacb37d4b14e\"},{\"content\":{\"connectorIds\":[\"Out1\",\"Out2\",\"Out4\",\"Out3\",\"Out5\"],\"side\":\"RIGHT\"},\"type\":\"ConnectorPlacement.EquallySpacedRectSide\",\"uuid\":\"f03e67c3-9067-4270-99e4-3af62f53d6d4\"},{\"content\":{\"connectorIds\":[],\"side\":\"TOP\"},\"type\":\"ConnectorPlacement.EquallySpacedRectSide\",\"uuid\":\"95121101-a1f3-498e-9169-a50ee0e00c46\"}]},\"type\":\"ConnectorPlacement.EquallySpacedConnector\",\"uuid\":\"037076c6-6da9-4e6a-8e27-787cb4a9f20b\"}],\"packageUris\":[\"http://schema.mathworks.com/mf0/Connector/R2020b\"],\"version\":\"1.0\"}"
  FL_boREQ_MainHV_ON_PLUS : Outport
  FL_boREQ_MainHV_ON_MINUS : Outport  Port=2
  FL_boMainHV_Minus_Welded : Outport  Port=3
  FL_boMainHV_Plus_Welded : Outport  Port=4
  FL_u8WeldingDetection_Status : Outport  Port=5
  wires:
  Chart_WeldingDetection/4(REQ_MainHV_ON_PLUS) -> FL_boREQ_MainHV_ON_PLUS/1
  Chart_WeldingDetection/3(REQ_MainHV_ON_MINUS) -> FL_boREQ_MainHV_ON_MINUS/1
  LoadVtg/1 -> Chart_WeldingDetection/1(LoadVtg)
  SystemVtg/1 -> Chart_WeldingDetection/2(SystemVtg)
  FL_boMainHV_WeldingCheckEnable/1 -> Chart_WeldingDetection/3(In)
  Chart_WeldingDetection/1(MainHV_Minus_Welded) -> FL_boMainHV_Minus_Welded/1
  Chart_WeldingDetection/2(MainHV_Plus_Welded) -> FL_boMainHV_Plus_Welded/1
  Chart_WeldingDetection/5(WeldingDetection_Status) -> FL_u8WeldingDetection_Status/1

== system ChiefMaster_TTC580/ChiefMaster/Flow Logic/BDU Control/BDUSystem/Subsystem3 ==
  FL_boREQ_DC_ON : Inport
  IT_boHW_DCHV_Plus_FB : Inport  Port=2
  IT_boHW_DCHV_Minus_FB : Inport  Port=3
  CMShutdown : Inport  Port=4
  Chart_Main_MinMAx_Status : libCM/Chart_Main_MinMAx_Status  SystemSampleTime=-1  VariantActivationTime=update diagram  Latency=0  AutoFrameSizeCalculation=off
      settings: PortSchema="{\"entries\":[{\"content\":{\"sides\":[{\"content\":{\"connectorIds\":[\"In1\",\"In2\",\"In4\",\"In3\"]},\"type\":\"ConnectorPlacement.EquallySpacedRectSide\",\"uuid\":\"af513ad7-882d-44ca-bd16-f13375ad0cc7\"},{\"content\":{\"connectorIds\":[\"Out1\"],\"side\":\"RIGHT\"},\"type\":\"ConnectorPlacement.EquallySpacedRectSide\",\"uuid\":\"1e07241b-ff1c-4b1c-99ea-8f556d1f4bde\"},{\"content\":{\"connectorIds\":[],\"side\":\"TOP\"},\"type\":\"ConnectorPlacement.EquallySpacedRectSide\",\"uuid\":\"c2fbf455-7245-4f9b-917b-4eed34a267cf\"}]},\"type\":\"ConnectorPlacement.EquallySpacedConnector\",\"uuid\":\"56193be1-d801-449e-8417-1819ff958dca\"}],\"packageUris\":[\"http://schema.mathworks.com/mf0/Connector/R2020b\"],\"version\":\"1.0\"}"
  Chart_Main_MinMAx_Status1 : libCM/Chart_Main_MinMAx_Status  SystemSampleTime=-1  VariantActivationTime=update diagram  Latency=0  AutoFrameSizeCalculation=off
      settings: PortSchema="{\"entries\":[{\"content\":{\"sides\":[{\"content\":{\"connectorIds\":[\"In1\",\"In2\",\"In4\",\"In3\"]},\"type\":\"ConnectorPlacement.EquallySpacedRectSide\",\"uuid\":\"af513ad7-882d-44ca-bd16-f13375ad0cc7\"},{\"content\":{\"connectorIds\":[\"Out1\"],\"side\":\"RIGHT\"},\"type\":\"ConnectorPlacement.EquallySpacedRectSide\",\"uuid\":\"1e07241b-ff1c-4b1c-99ea-8f556d1f4bde\"},{\"content\":{\"connectorIds\":[],\"side\":\"TOP\"},\"type\":\"ConnectorPlacement.EquallySpacedRectSide\",\"uuid\":\"c2fbf455-7245-4f9b-917b-4eed34a267cf\"}]},\"type\":\"ConnectorPlacement.EquallySpacedConnector\",\"uuid\":\"56193be1-d801-449e-8417-1819ff958dca\"}],\"packageUris\":[\"http://schema.mathworks.com/mf0/Connector/R2020b\"],\"version\":\"1.0\"}"
  Constant2 : Constant  Value=MainHV_StatusDelay
  FL_u8DCHV_Minus_Status : Outport
  FL_u8DCHV_Plus_Status : Outport  Port=2
  wires:
  Constant2/1 -> Chart_Main_MinMAx_Status1/3, Chart_Main_MinMAx_Status/3
  Chart_Main_MinMAx_Status1/1 -> FL_u8DCHV_Plus_Status/1  "FL_u8DCHV_Plus_Status"
  Chart_Main_MinMAx_Status/1 -> FL_u8DCHV_Minus_Status/1  "FL_u8DCHV_Minus_Status"
  FL_boREQ_DC_ON/1 -> Chart_Main_MinMAx_Status1/1, Chart_Main_MinMAx_Status/1
  IT_boHW_DCHV_Minus_FB/1 -> Chart_Main_MinMAx_Status/2
  CMShutdown/1 -> Chart_Main_MinMAx_Status1/4, Chart_Main_MinMAx_Status/4
  IT_boHW_DCHV_Plus_FB/1 -> Chart_Main_MinMAx_Status1/2

== system ChiefMaster_TTC580/ChiefMaster/Flow Logic/System Status/CurrentPrognosis/Subsystem ==
  <IP_boBMS_HV_REL_ON_BB1> : Inport
  <IP_boBMS_HV_REL_ON_BB2> : Inport  Port=2
  <IP_boBMS_HV_REL_ON_BB3> : Inport  Port=3
  <IP_sBMS_Current_BB1> : Inport  Port=4
  <IP_sBMS_Current_BB2> : Inport  Port=5
  <IP_sBMS_Current_BB3> : Inport  Port=6
  AND : Logic  Inputs=3  AllPortsSameDT=off  OutDataTypeStr=boolean
  AND1 : Logic  Inputs=3  AllPortsSameDT=off  OutDataTypeStr=boolean
  AND2 : Logic  Inputs=3  AllPortsSameDT=off  OutDataTypeStr=boolean
  Compare To Constant : simulink/Logic and Bit Operations/Compare To Constant  relop=>=  const=15  OutDataTypeStr=boolean
  Compare To Constant1 : simulink/Logic and Bit Operations/Compare To Constant  relop=>=  const=15  OutDataTypeStr=boolean
  Compare To Constant2 : simulink/Logic and Bit Operations/Compare To Constant  relop=>=  const=15  OutDataTypeStr=boolean
  Compare To Constant3 : simulink/Logic and Bit Operations/Compare To Constant  relop=>=  const=10  OutDataTypeStr=boolean
  Compare To Constant4 : simulink/Logic and Bit Operations/Compare To Constant  relop=>=  const=10  OutDataTypeStr=boolean
  Compare To Constant5 : simulink/Logic and Bit Operations/Compare To Constant  relop=>=  const=10  OutDataTypeStr=boolean
  Compare To Constant6 : simulink/Logic and Bit Operations/Compare To Constant  relop=>=  const=5  OutDataTypeStr=boolean
  Compare To Constant7 : simulink/Logic and Bit Operations/Compare To Constant  relop=>=  const=5  OutDataTypeStr=boolean
  Compare To Constant8 : simulink/Logic and Bit Operations/Compare To Constant  relop=>=  const=5  OutDataTypeStr=boolean
  Constant : Constant  Value=65535
  Constant1 : Constant  Value=65535
  Constant2 : Constant  Value=65535
  Constant3 : Constant  Value=CurrentReductionConstant_Lvl2  OutDataTypeStr=single
  Constant4 : Constant  Value=CurrentReductionConstant_Lvl1  OutDataTypeStr=single
  Constant5 : Constant  Value=CurrentReductionConstant_Lvl3  OutDataTypeStr=single
  Constant6 : Constant  Value=CurrentReductionConstant_Lvl0  OutDataTypeStr=single
  Switch{,1..5} (6 alike) : Switch  Criteria=u2 > Threshold  SaturateOnIntegerOverflow=off  InputSameDT=off
  CurrentReductionConstant : Outport
  wires:
  Constant6/1 -> Switch5/3
  Constant4/1 -> Switch5/1
  Switch5/1 -> Switch4/3
  AND2/1 -> Switch5/2
  Compare To Constant6/1 -> AND2/1
  Compare To Constant7/1 -> AND2/2
  Compare To Constant8/1 -> AND2/3
  Constant3/1 -> Switch4/1
  Switch4/1 -> Switch3/3
  AND1/1 -> Switch4/2
  Compare To Constant5/1 -> AND1/3
  Compare To Constant4/1 -> AND1/2
  Compare To Constant3/1 -> AND1/1
  Switch3/1 -> CurrentReductionConstant/1
  AND/1 -> Switch3/2
  Switch2/1 -> Compare To Constant2/1, Compare To Constant5/1, Compare To Constant8/1
  Compare To Constant2/1 -> AND/3
  Switch1/1 -> Compare To Constant1/1, Compare To Constant4/1, Compare To Constant7/1
  Compare To Constant1/1 -> AND/2
  Compare To Constant/1 -> AND/1
  Switch/1 -> Compare To Constant/1, Compare To Constant3/1, Compare To Constant6/1
  <IP_boBMS_HV_REL_ON_BB3>/1 -> Switch2/2
  <IP_sBMS_Current_BB3>/1 -> Switch2/1
  Constant2/1 -> Switch2/3
  <IP_sBMS_Current_BB2>/1 -> Switch1/1
  <IP_boBMS_HV_REL_ON_BB2>/1 -> Switch1/2
  Constant1/1 -> Switch1/3
  Constant/1 -> Switch/3
  <IP_sBMS_Current_BB1>/1 -> Switch/1
  <IP_boBMS_HV_REL_ON_BB1>/1 -> Switch/2
  Constant5/1 -> Switch3/1

== system ChiefMaster_TTC580/ChiefMaster/Flow Logic/System Status/EmergencySD/Emergency_Switch_Control ==
  reset : Inport
  IT_boEmergencySwitch_NC_S2 : Inport  Port=2
  IT_boVS_EmergencySwitch_NO_S1 : Inport  Port=3
  AND : Logic  Inputs=4  AllPortsSameDT=off  OutDataTypeStr=boolean
  EmergencySwitch_Input_Delay : Stateflow chart  TreatAsAtomicUnit=on
  EmergencySwitch_Input_Delay1 : Stateflow chart  TreatAsAtomicUnit=on
  fcn_EmergencyButtonState : Subsystem  Commented=on  TreatAsAtomicUnit=on  ReferencedSubsystem=fcn_EmergencyStopState
      settings: RTWFcnNameOpts=Use subsystem name  RTWFileNameOpts=Use subsystem name
  FL_u8VS_EmergencyStopState : Outport
  wires:
  AND/1 -> FL_u8VS_EmergencyStopState/1
  IT_boVS_EmergencySwitch_NO_S1/1 -> EmergencySwitch_Input_Delay1/1(IP_boVS_EmergensySwitch)
  EmergencySwitch_Input_Delay/1(out) -> AND/3, AND/2
  IT_boEmergencySwitch_NC_S2/1 -> EmergencySwitch_Input_Delay/1(IP_boVS_EmergensySwitch)
  reset/1 -> AND/4
  EmergencySwitch_Input_Delay1/1(out) -> AND/1

== system ChiefMaster_TTC580/ChiefMaster/Flow Logic/System Status/EmergencySD/HVIL_NOK ==
  boReset : Inport
  <IT_boHW_HVIL_BDU> : Inport  Port=2
  <IT_boHW_HVIL_Components> : Inport  Port=3
  <IT_boHW_HVIL_Battery> : Inport  Port=4
  Compare To Constant1 : simulink/Logic and Bit Operations/Compare To Constant  relop===  const=0  OutDataTypeStr=boolean
  Compare To Constant2 : simulink/Logic and Bit Operations/Compare To Constant  relop===  const=0  OutDataTypeStr=boolean
  Compare To Constant3 : simulink/Logic and Bit Operations/Compare To Constant  relop===  const=0  OutDataTypeStr=boolean
  Lib_SetDominantSwitch : Library_DataProcessing_v1_1/Lib_SetDominantSwitch  SystemSampleTime=-1  VariantActivationTime=update diagram  Latency=0  AutoFrameSizeCalculation=off
  Lib_SetDominantSwitch1 : Library_DataProcessing_v1_1/Lib_SetDominantSwitch  SystemSampleTime=-1  VariantActivationTime=update diagram  Latency=0  AutoFrameSizeCalculation=off
  Lib_SetDominantSwitch2 : Library_DataProcessing_v1_1/Lib_SetDominantSwitch  SystemSampleTime=-1  VariantActivationTime=update diagram  Latency=0  AutoFrameSizeCalculation=off
  OR : Logic  Operator=OR  Inputs=3  AllPortsSameDT=off  OutDataTypeStr=boolean
  FL_boSS_HVIL_NOK : Outport
  wires:
  Compare To Constant1/1 -> Lib_SetDominantSwitch/1
  Lib_SetDominantSwitch2/1 -> OR/3
  <IT_boHW_HVIL_Battery>/1 -> Compare To Constant3/1
  Lib_SetDominantSwitch1/1 -> OR/2
  boReset/1 -> Lib_SetDominantSwitch2/2, Lib_SetDominantSwitch1/2, Lib_SetDominantSwitch/2
  Compare To Constant3/1 -> Lib_SetDominantSwitch2/1
  Compare To Constant2/1 -> Lib_SetDominantSwitch1/1
  Lib_SetDominantSwitch/1 -> OR/1
  <IT_boHW_HVIL_BDU>/1 -> Compare To Constant1/1
  <IT_boHW_HVIL_Components>/1 -> Compare To Constant2/1
  OR/1 -> FL_boSS_HVIL_NOK/1  "FL_boSS_HVIL_NOK"

== system ChiefMaster_TTC580/ChiefMaster/Flow Logic/System Status/SDError/BDU_Error ==
  Main_REL_Databus : Inport
  Bus Selector1 : BusSelector  OutputSignals=FL_u8MainHV_Minus_Status,FL_u8MainHV_Plus_Status,FL_u8Precharge_Status
  Compare To Constant6 : simulink/Logic and Bit Operations/Compare To Constant  relop===  const=3  OutDataTypeStr=boolean
  Compare To Constant7 : simulink/Logic and Bit Operations/Compare To Constant  relop===  const=3  OutDataTypeStr=boolean
  Compare To Constant8 : simulink/Logic and Bit Operations/Compare To Constant  relop===  const=2  OutDataTypeStr=boolean
  OR1 : Logic  Operator=OR  Inputs=3  AllPortsSameDT=off  OutDataTypeStr=boolean
  Unit Delay : UnitDelay  SampleTime=-1  HasFrameUpgradeWarning=on
  Unit Delay1 : UnitDelay  SampleTime=-1  HasFrameUpgradeWarning=on
  Unit Delay2 : UnitDelay  SampleTime=-1  HasFrameUpgradeWarning=on
  BDU_Error : Outport
  wires:
  Main_REL_Databus/1 -> Bus Selector1/1
  Bus Selector1/2 -> Unit Delay1/1  "<FL_u8MainHV_Plus_Status>"
  Unit Delay1/1 -> Compare To Constant7/1
  Compare To Constant6/1 -> OR1/1
  Bus Selector1/1 -> Unit Delay/1  "<FL_u8MainHV_Minus_Status>"
  Bus Selector1/3 -> Unit Delay2/1  "<FL_u8Precharge_Status>"
  Compare To Constant8/1 -> OR1/3
  OR1/1 -> BDU_Error/1
  Unit Delay/1 -> Compare To Constant6/1
  Compare To Constant7/1 -> OR1/2
  Unit Delay2/1 -> Compare To Constant8/1

== system ChiefMaster_TTC580/ChiefMaster/Flow Logic/System Status/SDError/IMD_Error ==
  BatteryPackSignals : Inport
  AND1 : Logic  AllPortsSameDT=off  OutDataTypeStr=boolean
  AND2 : Logic  AllPortsSameDT=off  OutDataTypeStr=boolean
  AND3 : Logic  AllPortsSameDT=off  OutDataTypeStr=boolean
  Bus Selector1 : BusSelector  OutputSignals=IT_BatterySignal_Databus.IT_boBMS_IMD_Active_BB1,IT_BatterySignal_Databus.IT_boBMS_IMD_Active_BB2,IT_BatterySignal_Databus.IT_boBMS_IMD_Active_BB3,IT_BatterySignal_Databus.IT_boBMS_HV_REL_ON_BB1,IT_BatterySignal_Databus.IT_boBMS_HV_REL_ON_BB2,IT_BatterySignal_Databus.IT_boBMS_HV_REL_ON_BB3
  Constant : Constant  OutDataTypeStr=boolean
  GreaterThan : RelationalOperator  Operator=>  OutDataTypeStr=boolean  RndMeth=Simplest  InputSameDT=off
  OR : Logic  Operator=OR  Inputs=3  AllPortsSameDT=off  OutDataTypeStr=boolean
  Sum : Sum  Inputs=+++
  Terminator : Terminator
  IMD_Error : Outport
  wires:
  Sum/1 -> GreaterThan/1
  AND3/1 -> Sum/3
  Bus Selector1/3 -> AND3/1  "<IT_boBMS_IMD_Active_BB3>"
  AND2/1 -> Sum/2
  AND1/1 -> Sum/1
  Bus Selector1/2 -> AND2/1  "<IT_boBMS_IMD_Active_BB2>"
  Bus Selector1/1 -> AND1/1  "<IT_boBMS_IMD_Active_BB1>"
  GreaterThan/1 -> IMD_Error/1
  Bus Selector1/6 -> AND3/2, OR/3  "<IT_boBMS_HV_REL_ON_BB3>"
  Bus Selector1/4 -> OR/1, AND1/2  "<IT_boBMS_HV_REL_ON_BB1>"
  Bus Selector1/5 -> AND2/2, OR/2  "<IT_boBMS_HV_REL_ON_BB2>"
  OR/1 -> Terminator/1
  BatteryPackSignals/1 -> Bus Selector1/1
  Constant/1 -> GreaterThan/2

== system ChiefMaster_TTC580/ChiefMaster/Flow Logic/System Status/SDError/IMD_SD ==
  BatteryPackSignals : Inport
  AND : Logic  Inputs=3  AllPortsSameDT=off  OutDataTypeStr=boolean
  AND1 : Logic  Inputs=3  AllPortsSameDT=off  OutDataTypeStr=boolean
  AND2 : Logic  Inputs=3  AllPortsSameDT=off  OutDataTypeStr=boolean
  Bus Selector1 : BusSelector  OutputSignals=IT_BatterySignal_Databus.IT_boBMS_InsulationReadyOK_B1,IT_BatterySignal_Databus.IT_boBMS_InsulationSDError_B1,IT_BatterySignal_Databus.IT_boBMS_IMD_Active_BB1,IT_BatterySignal_Databus.IT_boBMS_HV_REL_ON_BB1,IT_BatterySignal_Databus.IT_boBMS_InsulationReadyOK_B2,IT_BatterySignal_Databus.IT_boBMS_InsulationSDError_B2,IT_BatterySignal_Databus.IT_boBMS_IMD_Active_BB2,IT_BatterySignal_Databus.IT_boBMS_HV_REL_ON_BB2,IT_BatterySignal_Databus.IT_boBMS_InsulationReadyOK_B3,IT_BatterySignal_Databus.IT_boBMS_InsulationSDError_B3,IT_BatterySignal_Databus.IT_boBMS_IMD_Active_BB3,IT_BatterySignal_Databus.IT_boBMS_HV_REL_ON_BB3
  Chart : Stateflow chart  TreatAsAtomicUnit=on
  Chart1 : Stateflow chart  TreatAsAtomicUnit=on
  Chart2 : Stateflow chart  TreatAsAtomicUnit=on
  OR : Logic  Operator=OR  Inputs=3  AllPortsSameDT=off  OutDataTypeStr=boolean
  IMD_SDError : Outport
  wires:
  Chart2/1(IMD_Error) -> AND2/1
  Chart1/1(IMD_Error) -> AND1/1
  Bus Selector1/11 -> AND2/2  "<IT_boBMS_IMD_Active_BB3>"
  Bus Selector1/7 -> AND1/2  "<IT_boBMS_IMD_Active_BB2>"
  Bus Selector1/10 -> Chart2/2(IP_boBMS_InsulationSDError)  "<IT_boBMS_InsulationSDError_B3>"
  Bus Selector1/6 -> Chart1/2(IP_boBMS_InsulationSDError)  "<IT_boBMS_InsulationSDError_B2>"
  Bus Selector1/9 -> Chart2/1(IP_boBMS_InsulationReadyOK)  "<IT_boBMS_InsulationReadyOK_B3>"
  Bus Selector1/5 -> Chart1/1(IP_boBMS_InsulationReadyOK)  "<IT_boBMS_InsulationReadyOK_B2>"
  Chart/1(IMD_Error) -> AND/1
  Bus Selector1/1 -> Chart/1(IP_boBMS_InsulationReadyOK)  "<IT_boBMS_InsulationReadyOK_B1>"
  AND2/1 -> OR/3
  AND1/1 -> OR/2
  AND/1 -> OR/1
  Bus Selector1/3 -> AND/2  "<IT_boBMS_IMD_Active_BB1>"
  Bus Selector1/2 -> Chart/2(IP_boBMS_InsulationSDError)  "<IT_boBMS_InsulationSDError_B1>"
  OR/1 -> IMD_SDError/1  "IMD_SDError"
  BatteryPackSignals/1 -> Bus Selector1/1
  Bus Selector1/4 -> AND/3  "<IT_boBMS_HV_REL_ON_BB1>"
  Bus Selector1/8 -> AND1/3  "<IT_boBMS_HV_REL_ON_BB2>"
  Bus Selector1/12 -> AND2/3  "<IT_boBMS_HV_REL_ON_BB3>"
